simulink model "ctrl_typeA"  (R2016b)
settings: Solver=ode45  StartTime=0.0  StopTime=12.0  RelTol=1e-3  EnableMultiTasking=on
undefined symbols (not defined in the file): cMat_BF, cMat_IM, cMat_MN, cMat_TM, gain_actBFGAS, gain_actBFL, gain_actBFP, gain_actBFR, gain_actBFT, gain_actBFV, gain_actBFY, gain_actF0GAS, gain_actF1GAS, gain_actF2GAS, gain_actF3GAS, gain_actIML, gain_actIMP, gain_actIMR, gain_actIMT, gain_actIMV, gain_actIMY, gain_actIPL, gain_actIPT, gain_actIPY, gain_actMNL, gain_actMNP, gain_actMNR, gain_actMNT, gain_actMNV, gain_actMNY, gain_actTML, gain_actTMP, gain_actTMY, gainBFGAS, gainBFL, gainBFP, gainBFR, gainBFT, gainBFV, gainBFY, gainF0GAS, gainF1GAS, gainF2GAS, gainF3GAS, gainHieBFP, gainHieBFR, gainHieBFY, gainHieIML, gainHieIMP, gainHieIMY, gainHieIPL, gainHieIPY, gainHieMNL, gainHieMNP, gainHieMNY, gainIML, gainIMP, gainIMR, gainIMT, gainIMV ... (+24)
libraries: cstblocks x54
(part 1 of 2)
settings Model: Creator=kokioktm  LastModifiedBy=miyo
settings DataIOCC: LimitDataPoints=on  SaveFormat=Array
settings OptimizationCC: LifeSpan=inf
settings DebuggingCC: SFUnexpectedBacktrackingDiag=warning  SFNoUnconditionalDefaultTransitionDiag=warning  SFExecutionAtInitializationDiag=none
settings HardwareCC: ProdBitPerPointer=32  ProdBitPerSizeT=32  ProdBitPerPtrDiffT=32  ProdLargestAtomicFloat=None  ProdIntDivRoundTo=Undefined  ProdEndianess=Unspecified  ProdWordSize=32  ProdHWDeviceType=32-bit Generic
settings ModelReferenceCC: PropagateSignalLabelsOutOfModel=off
settings GRTTargetCC: TargetLangStandard=C89/C90 (ANSI)  GeneratePreprocessorConditionals=Disable all
settings ConfigComp: CovMetricSettings=dw  CovHtmlReporting=on  CovSaveCumulativeToWorkspaceVar=on  CovSaveSingleToWorkspaceVar=on  CovExternalEMLEnable=off  CovSFcnEnable=off

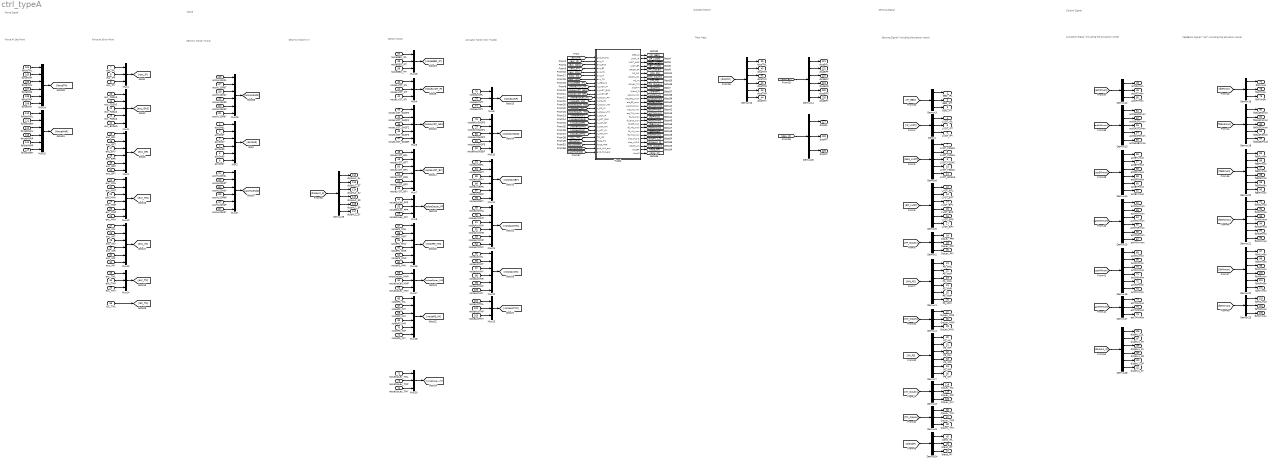
== system ctrl_typeA ==
  note: Actuator Noise
      | (only TypeA)
  note: Force
      | at Error Point
  note: Sensor Noise
  note: Seismic Noise
      | (m/s/s)
  note: Noise
  note: Seismic Noise
      | (m)
  note: Sensing Signal
      | (including the
      | sensor noise)
  note: FeedBack Signal
      | ("not" including the
      | actuation noise)
  note: Actuation Signal
      | (including the
      | actuation noise)
  note: Force
      | At Set Point
  note: Force Signal
  note: Control Signal
  note: Sensing Signal
  note: Test Mass
  note: Isolated Motion
  accGndL : Inport
  accGndT : Inport  Port=2
  accGndV : Inport  Port=3
  accGndR : Inport  Port=4
  accGndP : Inport  Port=5
  accGndY : Inport  Port=6
  exc_IPL : Inport  Port=7
  exc_IPT : Inport  Port=8
  exc_IPY : Inport  Port=9
  exc_F0GAS : Inport  Port=10
  exc_F1GAS : Inport  Port=11
  exc_F2GAS : Inport  Port=12
  exc_F3GAS : Inport  Port=13
  exc_BFGAS : Inport  Port=14
  exc_BFL : Inport  Port=15
  exc_BFT : Inport  Port=16
  exc_BFV : Inport  Port=17
  exc_BFR : Inport  Port=18
  exc_BFP : Inport  Port=19
  exc_BFY : Inport  Port=20
  exc_MNL : Inport  Port=21
  exc_MNT : Inport  Port=22
  exc_MNV : Inport  Port=23
  exc_MNR : Inport  Port=24
  exc_MNP : Inport  Port=25
  exc_MNY : Inport  Port=26
  exc_IML : Inport  Port=27
  exc_IMT : Inport  Port=28
  exc_IMV : Inport  Port=29
  exc_IMR : Inport  Port=30
  exc_IMP : Inport  Port=31
  exc_IMY : Inport  Port=32
  exc_TML : Inport  Port=33
  exc_TMP : Inport  Port=34
  exc_TMY : Inport  Port=35
  ISC_TML : Inport  Port=36
  noiseGEO_IPL : Inport  Port=37
  noiseGEO_IPT : Inport  Port=38
  noiseGEO_IPY : Inport  Port=39
  noiseLVDT_IPL : Inport  Port=40
  noiseLVDT_IPT : Inport  Port=41
  noiseLVDT_IPY : Inport  Port=42
  noiseLVDT_GASF0 : Inport  Port=43
  noiseLVDT_GASF1 : Inport  Port=44
  noiseLVDT_GASF2 : Inport  Port=45
  noiseLVDT_GASF3 : Inport  Port=46
  noiseLVDT_GASBF : Inport  Port=47
  noiseLVDT_BFL : Inport  Port=48
  noiseLVDT_BFT : Inport  Port=49
  noiseLVDT_BFV : Inport  Port=50
  noiseLVDT_BFR : Inport  Port=51
  noiseLVDT_BFP : Inport  Port=52
  noiseLVDT_BFY : Inport  Port=53
  noiseOpLev_PFR : Inport  Port=54
  noiseOpLev_PFP : Inport  Port=55
  noiseOpLev_PFY : Inport  Port=56
  noisePS_MNL : Inport  Port=57
  noisePS_MNT : Inport  Port=58
  noisePS_MNV : Inport  Port=59
  noisePS_MNR : Inport  Port=60
  noisePS_MNP : Inport  Port=61
  noisePS_MNY : Inport  Port=62
  noiseOpLev_MNR : Inport  Port=63
  noiseOpLev_MNP : Inport  Port=64
  noiseOpLev_MNY : Inport  Port=65
  noisePS_IML : Inport  Port=66
  noisePS_IMT : Inport  Port=67
  noisePS_IMV : Inport  Port=68
  noisePS_IMR : Inport  Port=69
  noisePS_IMP : Inport  Port=70
  noisePS_IMY : Inport  Port=71
  noiseOpLev_TML : Inport  Port=72
  noiseOpLev_TMP : Inport  Port=73
  noiseOpLev_TMY : Inport  Port=74
  noiseActIPL : Inport  Port=75
  noiseActIPT : Inport  Port=76
  noiseActIPY : Inport  Port=77
  noiseActGASF0 : Inport  Port=78
  noiseActGASF1 : Inport  Port=79
  noiseActGASF2 : Inport  Port=80
  noiseActGASF3 : Inport  Port=81
  noiseActGASBF : Inport  Port=82
  noiseActBFL : Inport  Port=83
  noiseActBFT : Inport  Port=84
  noiseActBFV : Inport  Port=85
  noiseActBFR : Inport  Port=86
  noiseActBFP : Inport  Port=87
  noiseActBFY : Inport  Port=88
  noiseActMNL : Inport  Port=89
  noiseActMNT : Inport  Port=90
  noiseActMNV : Inport  Port=91
  noiseActMNR : Inport  Port=92
  noiseActMNP : Inport  Port=93
  noiseActMNY : Inport  Port=94
  noiseActIML : Inport  Port=95
  noiseActIMT : Inport  Port=96
  noiseActIMV : Inport  Port=97
  noiseActIMR : Inport  Port=98
  noiseActIMP : Inport  Port=99
  noiseActIMY : Inport  Port=100
  noiseActTML : Inport  Port=101
  noiseActTMP : Inport  Port=102
  noiseActTMY : Inport  Port=103
  forceTML : Inport  Port=104
  forceTMT : Inport  Port=105
  forceTMV : Inport  Port=106
  forceTMR : Inport  Port=107
  forceTMP : Inport  Port=108
  forceTMY : Inport  Port=109
  forceMNRL : Inport  Port=110
  forceMNRT : Inport  Port=111
  forceMNRV : Inport  Port=112
  forceMNRR : Inport  Port=113
  forceMNRP : Inport  Port=114
  forceMNRY : Inport  Port=115
  accHL1GndL : Inport  Port=116
  accHL1GndT : Inport  Port=117
  accHL1GndV : Inport  Port=118
  accHL1GndR : Inport  Port=119
  accHL1GndP : Inport  Port=120
  accHL1GndY : Inport  Port=121
  accHL2GndL : Inport  Port=122
  accHL2GndT : Inport  Port=123
  accHL2GndV : Inport  Port=124
  accHL2GndR : Inport  Port=125
  accHL2GndP : Inport  Port=126
  accHL2GndY : Inport  Port=127
  Demux{,2..4,8..9,12,17..18,23..25} (12 alike) : Demux  Outputs=3
  Demux{1,5,7,10..11,14..16,20..22,28..29} (13 alike) : Demux  Outputs=6
  Demux13 : Demux  Outputs=5
  Demux19 : Demux  Outputs=5
  Demux6 : Demux  Outputs=5
  Mux{1,4,8..9,14..15,17,20,23} (9 alike) : Mux  Inputs=3
  Mux10 : Mux  Inputs=5
  Mux{2..3,7,11..13,16,18,21..22,24..27} (14 alike) : Mux  Inputs=6
  Mux5 : Mux  Inputs=5
  Mux6 : Mux  Inputs=5
  TypeA : Subsystem
  GEO_IPL : Outport
  GEO_IPT : Outport  Port=2
  GEO_IPY : Outport  Port=3
  LVDT_IPL : Outport  Port=4
  LVDT_IPT : Outport  Port=5
  LVDT_IPY : Outport  Port=6
  LVDT_F0GAS : Outport  Port=7
  LVDT_F1GAS : Outport  Port=8
  LVDT_F2GAS : Outport  Port=9
  LVDT_F3GAS : Outport  Port=10
  LVDT_BFGAS : Outport  Port=11
  LVDT_BFL : Outport  Port=12
  LVDT_BFT : Outport  Port=13
  LVDT_BFV : Outport  Port=14
  LVDT_BFR : Outport  Port=15
  LVDT_BFP : Outport  Port=16
  LVDT_BFY : Outport  Port=17
  OpLev_PFR : Outport  Port=18
  OpLev_PFP : Outport  Port=19
  OpLev_PFY : Outport  Port=20
  PS_MNL : Outport  Port=21
  PS_MNT : Outport  Port=22
  PS_MNV : Outport  Port=23
  PS_MNR : Outport  Port=24
  PS_MNP : Outport  Port=25
  PS_MNY : Outport  Port=26
  OpLev_MNR : Outport  Port=27
  OpLev_MNP : Outport  Port=28
  OpLev_MNY : Outport  Port=29
  PS_IML : Outport  Port=30
  PS_IMT : Outport  Port=31
  PS_IMV : Outport  Port=32
  PS_IMR : Outport  Port=33
  PS_IMP : Outport  Port=34
  PS_IMY : Outport  Port=35
  OpLev_TML : Outport  Port=36
  OpLev_TMP : Outport  Port=37
  OpLev_TMY : Outport  Port=38
  dispTML : Outport  Port=39
  dispTMT : Outport  Port=40
  dispTMV : Outport  Port=41
  dispTMR : Outport  Port=42
  dispTMP : Outport  Port=43
  dispTMY : Outport  Port=44
  blend_IPL : Outport  Port=45
  blend_IPT : Outport  Port=46
  blend_IPY : Outport  Port=47
  actIPLmon : Outport  Port=48
  actIPTmon : Outport  Port=49
  actIPYmon : Outport  Port=50
  actGASF0mon : Outport  Port=51
  actGASF1mon : Outport  Port=52
  actGASF2mon : Outport  Port=53
  actGASF3mon : Outport  Port=54
  actGASBFmon : Outport  Port=55
  actBFLmon : Outport  Port=56
  actBFTmon : Outport  Port=57
  actBFVmon : Outport  Port=58
  actBFRmon : Outport  Port=59
  actBFPmon : Outport  Port=60
  actBFYmon : Outport  Port=61
  actMNLmon : Outport  Port=62
  actMNTmon : Outport  Port=63
  actMNVmon : Outport  Port=64
  actMNRmon : Outport  Port=65
  actMNPmon : Outport  Port=66
  actMNYmon : Outport  Port=67
  actIMLmon : Outport  Port=68
  actIMTmon : Outport  Port=69
  actIMVmon : Outport  Port=70
  actIMRmon : Outport  Port=71
  actIMPmon : Outport  Port=72
  actIMYmon : Outport  Port=73
  actTMLmon : Outport  Port=74
  actTMPmon : Outport  Port=75
  actTMYmon : Outport  Port=76
  fbIPLmon : Outport  Port=77
  fbIPTmon : Outport  Port=78
  fbIPYmon : Outport  Port=79
  fbGASF0mon : Outport  Port=80
  fbGASF1mon : Outport  Port=81
  fbGASF2mon : Outport  Port=82
  fbGASF3mon : Outport  Port=83
  fbGASBFmon : Outport  Port=84
  fbBFLmon : Outport  Port=85
  fbBFTmon : Outport  Port=86
  fbBFVmon : Outport  Port=87
  fbBFRmon : Outport  Port=88
  fbBFPmon : Outport  Port=89
  fbBFYmon : Outport  Port=90
  fbMNLmon : Outport  Port=91
  fbMNTmon : Outport  Port=92
  fbMNVmon : Outport  Port=93
  fbMNRmon : Outport  Port=94
  fbMNPmon : Outport  Port=95
  fbMNYmon : Outport  Port=96
  fbIMLmon : Outport  Port=97
  fbIMTmon : Outport  Port=98
  fbIMVmon : Outport  Port=99
  fbIMRmon : Outport  Port=100
  fbIMPmon : Outport  Port=101
  fbIMYmon : Outport  Port=102
  fbTMLmon : Outport  Port=103
  fbTMPmon : Outport  Port=104
  fbTMYmon : Outport  Port=105
  dispHL1_3L : Outport  Port=106
  dispHL1_3T : Outport  Port=107
  dispHL1_3V : Outport  Port=108
  dispHL1_3R : Outport  Port=109
  dispHL1_3P : Outport  Port=110
  dispHL1_3Y : Outport  Port=111
  dispHL2_3L : Outport  Port=112
  dispHL2_3T : Outport  Port=113
  dispHL2_3V : Outport  Port=114
  dispHL2_3R : Outport  Port=115
  dispHL2_3P : Outport  Port=116
  dispHL2_3Y : Outport  Port=117
  OpLev_IML : Outport  Port=118
  OpLev_IMP : Outport  Port=119
  OpLev_IMY : Outport  Port=120
  dispBFL : Outport  Port=121
  dispBFT : Outport  Port=122
  dispBFV : Outport  Port=123
  dispBFR : Outport  Port=124
  dispBFP : Outport  Port=125
  dispBFY : Outport  Port=126
  dispIPL : Outport  Port=127
  dispIPT : Outport  Port=128
  dispIPY : Outport  Port=129
  wires:
  [accGnd] -> TypeA/1(gnd_2F_acc)
  accGndT/1 -> Mux2/2
  accGndL/1 -> Mux2/1
  accGndV/1 -> Mux2/3
  accGndR/1 -> Mux2/4
  accGndP/1 -> Mux2/5
  accGndY/1 -> Mux2/6
  Mux2/1 -> [accGnd]
  exc_IPL/1 -> Mux1/1
  exc_IPT/1 -> Mux1/2
  exc_IPY/1 -> Mux1/3
  Mux1/1 -> [exc_IP]
  [exc_IP] -> TypeA/2(exc_IP)
  exc_F0GAS/1 -> Mux5/1
  exc_F1GAS/1 -> Mux5/2
  exc_F2GAS/1 -> Mux5/3
  exc_F3GAS/1 -> Mux5/4
  exc_BFGAS/1 -> Mux5/5
  Mux5/1 -> [exc_GAS]
  [exc_GAS] -> TypeA/3(exc_GAS)
  exc_BFT/1 -> Mux3/2
  exc_BFL/1 -> Mux3/1
  exc_BFV/1 -> Mux3/3
  exc_BFR/1 -> Mux3/4
  exc_BFP/1 -> Mux3/5
  exc_BFY/1 -> Mux3/6
  Mux3/1 -> [exc_BF]
  [exc_BF] -> TypeA/4(exc_BF)
  TypeA/2(LVDT_IP) -> [IP_LVDT]
  TypeA/3(LVDT_GAS) -> [GAS_LVDT]
  TypeA/4(LVDT_BF) -> [BF_LVDT]
  TypeA/10(dispTM) -> [dispTM]
  TypeA/5(OPLEV_PF) -> [PF_OpLev]
  [IP_LVDT] -> Demux/1
  Demux/1 -> LVDT_IPL/1
  Demux/2 -> LVDT_IPT/1
  Demux/3 -> LVDT_IPY/1
  [GAS_LVDT] -> Demux6/1
  Demux6/1 -> LVDT_F0GAS/1
  Demux6/2 -> LVDT_F1GAS/1
  Demux6/3 -> LVDT_F2GAS/1
  Demux6/4 -> LVDT_F3GAS/1
  Demux6/5 -> LVDT_BFGAS/1
  [BF_LVDT] -> Demux5/1
  Demux5/1 -> LVDT_BFL/1
  Demux5/2 -> LVDT_BFT/1
  Demux5/3 -> LVDT_BFV/1
  Demux5/4 -> LVDT_BFR/1
  Demux5/5 -> LVDT_BFP/1
  Demux5/6 -> LVDT_BFY/1
  Demux1/1 -> PS_MNL/1
  Demux1/2 -> PS_MNT/1
  Demux1/3 -> PS_MNV/1
  Demux1/4 -> PS_MNR/1
  Demux1/5 -> PS_MNP/1
  Demux1/6 -> PS_MNY/1
  [MN_PS] -> Demux1/1
  [PF_OpLev] -> Demux2/1
  Demux2/2 -> OpLev_PFP/1
  Demux2/3 -> OpLev_PFY/1
  noiseLVDT_IPL/1 -> Mux4/1
  noiseLVDT_IPT/1 -> Mux4/2
  noiseLVDT_IPY/1 -> Mux4/3
  Mux4/1 -> [noiseLVDT_IP]
  noiseLVDT_GASF0/1 -> Mux6/1
  noiseLVDT_GASF1/1 -> Mux6/2
  noiseLVDT_GASF2/1 -> Mux6/3
  noiseLVDT_GASF3/1 -> Mux6/4
  noiseLVDT_GASBF/1 -> Mux6/5
  Mux6/1 -> [noiseLVDT_GAS]
  noiseLVDT_BFT/1 -> Mux7/2
  noiseLVDT_BFL/1 -> Mux7/1
  noiseLVDT_BFV/1 -> Mux7/3
  noiseLVDT_BFR/1 -> Mux7/4
  noiseLVDT_BFP/1 -> Mux7/5
  noiseLVDT_BFY/1 -> Mux7/6
  Mux7/1 -> [noiseLVDT_BF]
  noiseOpLev_PFR/1 -> Mux8/1
  noiseOpLev_PFP/1 -> Mux8/2
  Mux8/1 -> [noiseOpLev_PF]
  [noiseLVDT_IP] -> TypeA/9(n_LVDT_IP)
  [noiseLVDT_GAS] -> TypeA/10(n_LVDT_GAS)
  [noiseOpLev_PF] -> TypeA/12(n_OpLev_PF)
  [noiseLVDT_BF] -> TypeA/11(n_LVDT_BF)
  noiseActIPL/1 -> Mux9/1
  noiseActIPT/1 -> Mux9/2
  noiseActIPY/1 -> Mux9/3
  Mux9/1 -> [noiseActIP]
  noiseActGASF0/1 -> Mux10/1
  noiseActGASF1/1 -> Mux10/2
  noiseActGASF2/1 -> Mux10/3
  noiseActGASF3/1 -> Mux10/4
  noiseActGASBF/1 -> Mux10/5
  Mux10/1 -> [noiseActGAS]
  noiseActBFT/1 -> Mux11/2
  noiseActBFL/1 -> Mux11/1
  noiseActBFV/1 -> Mux11/3
  noiseActBFR/1 -> Mux11/4
  noiseActBFP/1 -> Mux11/5
  noiseActBFY/1 -> Mux11/6
  Mux11/1 -> [noiseActBF]
  [noiseActGAS] -> TypeA/18(n_ACT_GAS)
  [noiseActBF] -> TypeA/19(n_ACT_BF)
  [noiseActIP] -> TypeA/17(n_ACT_IP)
  [exc_MN] -> TypeA/5(exc_MN)
  [exc_TM] -> TypeA/7(exc_TM)
  [exc_IM] -> TypeA/6(exc_IM)
  exc_MNT/1 -> Mux12/2
  exc_MNL/1 -> Mux12/1
  exc_MNV/1 -> Mux12/3
  exc_MNR/1 -> Mux12/4
  exc_MNP/1 -> Mux12/5
  exc_MNY/1 -> Mux12/6
  Mux12/1 -> [exc_MN]
  exc_IMT/1 -> Mux13/2
  exc_IML/1 -> Mux13/1
  exc_IMV/1 -> Mux13/3
  exc_IMR/1 -> Mux13/4
  exc_IMP/1 -> Mux13/5
  exc_IMY/1 -> Mux13/6
  Mux13/1 -> [exc_IM]
  exc_TML/1 -> Mux14/1
  exc_TMP/1 -> Mux14/2
  exc_TMY/1 -> Mux14/3
  Mux14/1 -> [exc_TM]
  noiseGEO_IPL/1 -> Mux15/1
  noiseGEO_IPT/1 -> Mux15/2
  noiseGEO_IPY/1 -> Mux15/3
  Mux15/1 -> [noiseGEO_IP]
  [noiseGEO_IP] -> TypeA/8(n_GEO_IP)
  noiseOpLev_PFY/1 -> Mux8/3
  noisePS_MNT/1 -> Mux16/2
  noisePS_MNL/1 -> Mux16/1
  noisePS_MNV/1 -> Mux16/3
  noisePS_MNR/1 -> Mux16/4
  noisePS_MNP/1 -> Mux16/5
  noisePS_MNY/1 -> Mux16/6
  Mux16/1 -> [noisePS_MN]
  noiseOpLev_MNR/1 -> Mux17/1
  noiseOpLev_MNP/1 -> Mux17/2
  Mux17/1 -> [noiseOpLev_MN]
  noiseOpLev_MNY/1 -> Mux17/3
  noisePS_IMT/1 -> Mux18/2
  noisePS_IML/1 -> Mux18/1
  noisePS_IMV/1 -> Mux18/3
  noisePS_IMR/1 -> Mux18/4
  noisePS_IMP/1 -> Mux18/5
  noisePS_IMY/1 -> Mux18/6
  Mux18/1 -> [noisePS_IM]
  noiseOpLev_TMP/1 -> Mux20/2
  noiseOpLev_TMY/1 -> Mux20/3
  Mux20/1 -> [noiseOpLev_TM]
  [noisePS_MN] -> TypeA/13(n_PS_MN)
  [noisePS_IM] -> TypeA/15(n_PS_IM)
  [noiseOpLev_MN] -> TypeA/14(n_OpLev_MN)
  [noiseOpLev_TM] -> TypeA/16(n_OpLev_TM)
  noiseActMNT/1 -> Mux21/2
  noiseActMNL/1 -> Mux21/1
  noiseActMNV/1 -> Mux21/3
  noiseActMNR/1 -> Mux21/4
  noiseActMNP/1 -> Mux21/5
  noiseActMNY/1 -> Mux21/6
  Mux21/1 -> [noiseActMN]
  noiseActIMT/1 -> Mux22/2
  noiseActIML/1 -> Mux22/1
  noiseActIMV/1 -> Mux22/3
  noiseActIMR/1 -> Mux22/4
  noiseActIMP/1 -> Mux22/5
  noiseActIMY/1 -> Mux22/6
  Mux22/1 -> [noiseActIM]
  noiseActTML/1 -> Mux23/1
  noiseActTMP/1 -> Mux23/2
  noiseActTMY/1 -> Mux23/3
  Mux23/1 -> [noiseActTM]
  forceTMT/1 -> Mux24/2
  forceTML/1 -> Mux24/1
  forceTMV/1 -> Mux24/3
  forceTMR/1 -> Mux24/4
  forceTMP/1 -> Mux24/5
  forceTMY/1 -> Mux24/6
  Mux24/1 -> [forceTM]
  ISC_TML/1 -> [ISC_TM]
  [noiseActMN] -> TypeA/20(n_ACT_MN)
  [noiseActTM] -> TypeA/22(n_ACT_TM)
  [noiseActIM] -> TypeA/21(n_ACT_IM)
  [forceTM] -> TypeA/24(force_TM)
  [ISC_TM] -> TypeA/23(TM_ISC)
  [IP_GEO] -> Demux3/1
  Demux3/1 -> GEO_IPL/1
  Demux3/2 -> GEO_IPT/1
  Demux3/3 -> GEO_IPY/1
  TypeA/1(GEO_IP) -> [IP_GEO]
  Demux2/1 -> OpLev_PFR/1
  TypeA/8(PS_IM) -> [IM_PS]
  TypeA/7(OPLEV_MN) -> [MN_OpLev]
  TypeA/6(PS_MN) -> [MN_PS]
  TypeA/9(OPLEV_TM) -> [TM_OpLev]
  TypeA/19(fb_GAS_mon) -> [fbGASmon]
  TypeA/13(act_GAS_mon) -> [actGASmon]
  TypeA/18(fb_IP_mon) -> [fbIPmon]
  TypeA/23(fb_TM_mon) -> [fbTMmon]
  TypeA/21(fb_MN_mon) -> [fbMNmon]
  TypeA/12(act_IP_mon) -> [actIPmon]
  TypeA/16(act_IM_mon) -> [actIMmon]
  TypeA/11(blend_IP) -> [blendIP]
  TypeA/22(fb_IM_mon) -> [fbIMmon]
  TypeA/15(act_MN_mon) -> [actMNmon]
  TypeA/17(act_TM_mon) -> [actTMmon]
  TypeA/14(act_BF_mon) -> [actBFmon]
  TypeA/20(fb_BF_mon) -> [fbBFmon]
  [MN_OpLev] -> Demux4/1
  Demux4/2 -> OpLev_MNP/1
  Demux4/3 -> OpLev_MNY/1
  Demux4/1 -> OpLev_MNR/1
  Demux7/1 -> PS_IML/1
  Demux7/2 -> PS_IMT/1
  Demux7/3 -> PS_IMV/1
  Demux7/4 -> PS_IMR/1
  Demux7/5 -> PS_IMP/1
  Demux7/6 -> PS_IMY/1
  [IM_PS] -> Demux7/1
  [TM_OpLev] -> Demux9/1
  Demux10/1 -> dispTML/1
  Demux10/2 -> dispTMT/1
  Demux10/3 -> dispTMV/1
  Demux10/4 -> dispTMR/1
  Demux10/5 -> dispTMP/1
  Demux10/6 -> dispTMY/1
  [dispTM] -> Demux10/1
  [actIPmon] -> Demux12/1
  Demux12/1 -> actIPLmon/1
  Demux12/2 -> actIPTmon/1
  Demux12/3 -> actIPYmon/1
  [actGASmon] -> Demux13/1
  Demux13/1 -> actGASF0mon/1
  Demux13/2 -> actGASF1mon/1
  Demux13/3 -> actGASF2mon/1
  Demux13/4 -> actGASF3mon/1
  Demux13/5 -> actGASBFmon/1
  [actBFmon] -> Demux14/1
  Demux14/1 -> actBFLmon/1
  Demux14/2 -> actBFTmon/1
  Demux14/3 -> actBFVmon/1
  Demux14/4 -> actBFRmon/1
  Demux14/5 -> actBFPmon/1
  Demux14/6 -> actBFYmon/1
  [actMNmon] -> Demux15/1
  Demux15/1 -> actMNLmon/1
  Demux15/2 -> actMNTmon/1
  Demux15/3 -> actMNVmon/1
  Demux15/4 -> actMNRmon/1
  Demux15/5 -> actMNPmon/1
  Demux15/6 -> actMNYmon/1
  [actIMmon] -> Demux16/1
  Demux16/1 -> actIMLmon/1
  Demux16/2 -> actIMTmon/1
  Demux16/3 -> actIMVmon/1
  Demux16/4 -> actIMRmon/1
  Demux16/5 -> actIMPmon/1
  Demux16/6 -> actIMYmon/1
  [actTMmon] -> Demux17/1
  Demux17/2 -> actTMPmon/1
  Demux17/3 -> actTMYmon/1
  Demux17/1 -> actTMLmon/1
  [fbIPmon] -> Demux18/1
  Demux18/1 -> fbIPLmon/1
  Demux18/2 -> fbIPTmon/1
  Demux18/3 -> fbIPYmon/1
  [fbGASmon] -> Demux19/1
  Demux19/1 -> fbGASF0mon/1
  Demux19/2 -> fbGASF1mon/1
  Demux19/3 -> fbGASF2mon/1
  Demux19/4 -> fbGASF3mon/1
  Demux19/5 -> fbGASBFmon/1
  [fbBFmon] -> Demux20/1
  Demux20/1 -> fbBFLmon/1
  Demux20/2 -> fbBFTmon/1
  Demux20/3 -> fbBFVmon/1
  Demux20/4 -> fbBFRmon/1
  Demux20/5 -> fbBFPmon/1
  Demux20/6 -> fbBFYmon/1
  [fbMNmon] -> Demux21/1
  Demux21/1 -> fbMNLmon/1
  Demux21/2 -> fbMNTmon/1
  Demux21/3 -> fbMNVmon/1
  Demux21/4 -> fbMNRmon/1
  Demux21/5 -> fbMNPmon/1
  Demux21/6 -> fbMNYmon/1
  [fbIMmon] -> Demux22/1
  Demux22/1 -> fbIMLmon/1
  Demux22/2 -> fbIMTmon/1
  Demux22/3 -> fbIMVmon/1
  Demux22/4 -> fbIMRmon/1
  Demux22/5 -> fbIMPmon/1
  Demux22/6 -> fbIMYmon/1
  [fbTMmon] -> Demux23/1
  Demux23/2 -> fbTMPmon/1
  Demux23/3 -> fbTMYmon/1
  Demux23/1 -> fbTMLmon/1
  Demux24/1 -> blend_IPL/1
  [blendIP] -> Demux24/1
  Demux24/2 -> blend_IPT/1
  Demux24/3 -> blend_IPY/1
  forceMNRR/1 -> Mux25/4
  forceMNRP/1 -> Mux25/5
  forceMNRL/1 -> Mux25/1
  forceMNRT/1 -> Mux25/2
  Mux25/1 -> [forceMNR]
  forceMNRV/1 -> Mux25/3
  forceMNRY/1 -> Mux25/6
  [forceMNR] -> TypeA/25(force_MNR)
  noiseOpLev_TML/1 -> Mux20/1
  Demux9/1 -> OpLev_TML/1
  Demux9/2 -> OpLev_TMP/1
  Demux9/3 -> OpLev_TMY/1
  TypeA/24(disp_HL1-3) -> [dispHL1_3]
  TypeA/25(disp_HL2-3) -> [dispHL2_3]
  Demux28/3 -> dispHL1_3V/1
  Demux28/1 -> dispHL1_3L/1
  Demux28/4 -> dispHL1_3R/1
  Demux28/2 -> dispHL1_3T/1
  Demux28/5 -> dispHL1_3P/1
  [dispHL1_3] -> Demux28/1
  Demux28/6 -> dispHL1_3Y/1
  Demux29/6 -> dispHL2_3Y/1
  [dispHL2_3] -> Demux29/1
  Demux29/1 -> dispHL2_3L/1
  Demux29/2 -> dispHL2_3T/1
  Demux29/5 -> dispHL2_3P/1
  Demux29/3 -> dispHL2_3V/1
  Demux29/4 -> dispHL2_3R/1
  accHL1GndP/1 -> Mux26/5
  accHL1GndL/1 -> Mux26/1
  accHL1GndR/1 -> Mux26/4
  accHL1GndY/1 -> Mux26/6
  Mux26/1 -> [accHLGnd1]
  accHL1GndV/1 -> Mux26/3
  accHL1GndT/1 -> Mux26/2
  [accHLGnd1] -> TypeA/26(gnd_HL1_acc)
  accHL2GndV/1 -> Mux27/3
  accHL2GndT/1 -> Mux27/2
  accHL2GndY/1 -> Mux27/6
  Mux27/1 -> [accHLGnd2]
  accHL2GndR/1 -> Mux27/4
  accHL2GndL/1 -> Mux27/1
  accHL2GndP/1 -> Mux27/5
  [accHLGnd2] -> TypeA/27(gnd_HL2_acc)
  TypeA/26(OPLEV_IM) -> [IM_OpLev]
  [IM_OpLev] -> Demux8/1
  Demux8/1 -> OpLev_IML/1
  Demux8/2 -> OpLev_IMP/1
  Demux8/3 -> OpLev_IMY/1
  TypeA/27(dispBF) -> [disp_BF]
  Demux11/1 -> dispBFL/1
  Demux11/2 -> dispBFT/1
  Demux11/3 -> dispBFV/1
  Demux11/4 -> dispBFR/1
  Demux11/5 -> dispBFP/1
  Demux11/6 -> dispBFY/1
  [disp_BF] -> Demux11/1
  TypeA/28(dispIP) -> [disp_IP]
  Demux25/1 -> dispIPL/1
  Demux25/2 -> dispIPT/1
  [disp_IP] -> Demux25/1
  Demux25/3 -> dispIPY/1

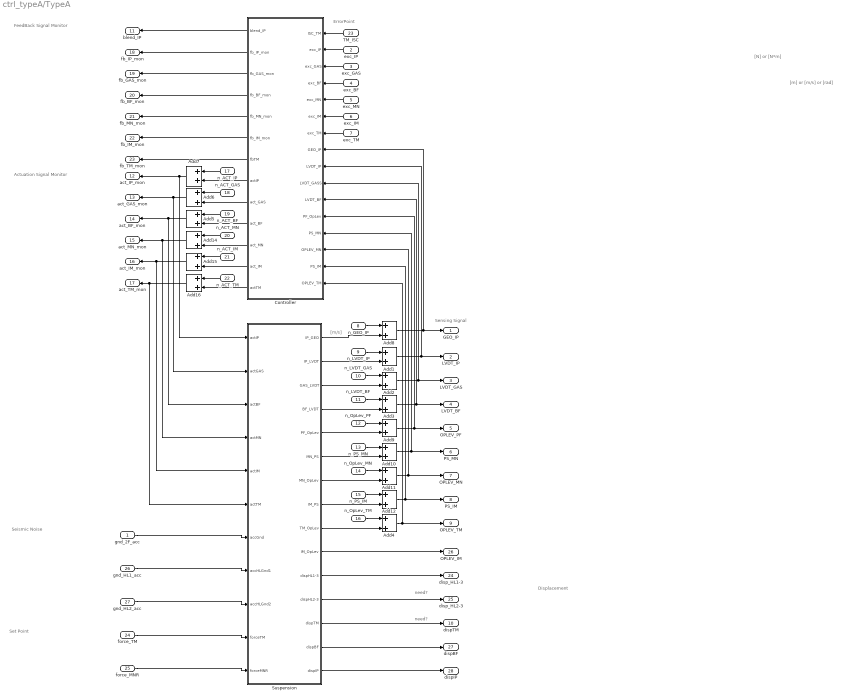
== system ctrl_typeA/TypeA ==
  note: [m] or [m/s] or [rad]
  note: [N] or [N*m]
  note: Sensing Signal
  note: Displacement
  note: Seismic
      | Noise
  note: Set Point
  note: Actuation Signal
      | Monitor
  note: FeedBack Signal
      | Monitor
  note: ErrorPoint
  note: [m/s]
  note: need?
  note: need?
  gnd_2F_acc : Inport
  exc_IP : Inport  Port=2
  exc_GAS : Inport  Port=3
  exc_BF : Inport  Port=4
  exc_MN : Inport  Port=5
  exc_IM : Inport  Port=6
  exc_TM : Inport  Port=7
  n_GEO_IP : Inport  Port=8
  n_LVDT_IP : Inport  Port=9
  n_LVDT_GAS : Inport  Port=10
  n_LVDT_BF : Inport  Port=11
  n_OpLev_PF : Inport  Port=12
  n_PS_MN : Inport  Port=13
  n_OpLev_MN : Inport  Port=14
  n_PS_IM : Inport  Port=15
  n_OpLev_TM : Inport  Port=16
  n_ACT_IP : Inport  Port=17
  n_ACT_GAS : Inport  Port=18
  n_ACT_BF : Inport  Port=19
  n_ACT_MN : Inport  Port=20
  n_ACT_IM : Inport  Port=21
  n_ACT_TM : Inport  Port=22
  TM_ISC : Inport  Port=23
  force_TM : Inport  Port=24
  force_MNR : Inport  Port=25
  gnd_HL1_acc : Inport  Port=26
  gnd_HL2_acc : Inport  Port=27
  Add{1..12,14..16} (15 alike) : Sum
  Controller : Subsystem
  Suspension : Subsystem
  GEO_IP : Outport
  LVDT_IP : Outport  Port=2
  LVDT_GAS : Outport  Port=3
  LVDT_BF : Outport  Port=4
  OPLEV_PF : Outport  Port=5
  PS_MN : Outport  Port=6
  OPLEV_MN : Outport  Port=7
  PS_IM : Outport  Port=8
  OPLEV_TM : Outport  Port=9
  dispTM : Outport  Port=10
  blend_IP : Outport  Port=11
  act_IP_mon : Outport  Port=12
  act_GAS_mon : Outport  Port=13
  act_BF_mon : Outport  Port=14
  act_MN_mon : Outport  Port=15
  act_IM_mon : Outport  Port=16
  act_TM_mon : Outport  Port=17
  fb_IP_mon : Outport  Port=18
  fb_GAS_mon : Outport  Port=19
  fb_BF_mon : Outport  Port=20
  fb_MN_mon : Outport  Port=21
  fb_IM_mon : Outport  Port=22
  fb_TM_mon : Outport  Port=23
  disp_HL1-3 : Outport  Port=24
  disp_HL2-3 : Outport  Port=25
  OPLEV_IM : Outport  Port=26
  dispBF : Outport  Port=27
  dispIP : Outport  Port=28
  wires:
  Add1/1 -> LVDT_IP/1, Controller/9(LVDT_IP)
  Add3/1 -> LVDT_BF/1, Controller/11(LVDT_BF)
  Add2/1 -> LVDT_GAS/1, Controller/10(LVDT_GASS)
  Suspension/13(dispTM) -> dispTM/1
  Add7/1 -> act_IP_mon/1, Suspension/1(actIP)
  Add5/1 -> act_BF_mon/1, Suspension/3(actBF)
  Add4/1 -> OPLEV_TM/1, Controller/16(OPLEV_TM)
  gnd_2F_acc/1 -> Suspension/7(accGnd)
  Add6/1 -> act_GAS_mon/1, Suspension/2(actGAS)
  exc_GAS/1 -> Controller/3(exc_GAS)
  exc_IP/1 -> Controller/2(exc_IP)
  exc_BF/1 -> Controller/4(exc_BF)
  Controller/4(fb_BF_mon) -> fb_BF_mon/1
  Controller/2(fb_IP_mon) -> fb_IP_mon/1
  Controller/3(fb_GAS_mon) -> fb_GAS_mon/1
  Suspension/2(IP_LVDT) -> Add1/2
  Suspension/3(GAS_LVDT) -> Add2/2
  Suspension/4(BF_LVDT) -> Add3/2
  Suspension/9(TM_OpLev) -> Add4/2
  n_LVDT_IP/1 -> Add1/1
  n_LVDT_GAS/1 -> Add2/1
  n_LVDT_BF/1 -> Add3/1
  n_OpLev_TM/1 -> Add4/1
  Controller/10(act_BF) -> Add5/2
  Controller/8(actIP) -> Add7/2
  Controller/9(act_GAS) -> Add6/2
  n_ACT_IP/1 -> Add7/1
  n_ACT_GAS/1 -> Add6/1
  n_ACT_BF/1 -> Add5/1
  Add8/1 -> GEO_IP/1, Controller/8(GEO_IP)
  n_GEO_IP/1 -> Add8/1
  Suspension/1(IP_GEO) -> Add8/2
  n_OpLev_PF/1 -> Add9/1
  Suspension/5(PF_OpLev) -> Add9/2
  Add9/1 -> OPLEV_PF/1, Controller/12(PF_OpLev)
  n_PS_MN/1 -> Add10/1
  Add10/1 -> PS_MN/1, Controller/13(PS_MN)
  n_OpLev_MN/1 -> Add11/1
  Add11/1 -> OPLEV_MN/1, Controller/14(OPLEV_MN)
  n_PS_IM/1 -> Add12/1
  Add12/1 -> PS_IM/1, Controller/15(PS_IM)
  Suspension/7(MN_OpLev) -> Add11/2
  Suspension/6(MN_PS) -> Add10/2
  Suspension/8(IM_PS) -> Add12/2
  exc_MN/1 -> Controller/5(exc_MN)
  exc_TM/1 -> Controller/7(exc_TM)
  exc_IM/1 -> Controller/6(exc_IM)
  TM_ISC/1 -> Controller/1(ISC_TM)
  n_ACT_MN/1 -> Add14/1
  Add14/1 -> act_MN_mon/1, Suspension/4(actMN)
  Controller/11(act_MN) -> Add14/2
  n_ACT_IM/1 -> Add15/1
  Add15/1 -> act_IM_mon/1, Suspension/5(actIM)
  Controller/12(act_IM) -> Add15/2
  n_ACT_TM/1 -> Add16/1
  Add16/1 -> act_TM_mon/1, Suspension/6(actTM)
  Controller/13(actTM) -> Add16/2
  Controller/1(blend_IP) -> blend_IP/1
  Controller/7(fbTM) -> fb_TM_mon/1
  Controller/5(fb_MN_mon) -> fb_MN_mon/1
  Controller/6(fb_IM_mon) -> fb_IM_mon/1
  force_TM/1 -> Suspension/10(forceTM)
  force_MNR/1 -> Suspension/11(forceMNR)
  Suspension/11(dispHL1-3) -> disp_HL1-3/1
  Suspension/12(dispHL2-3) -> disp_HL2-3/1
  gnd_HL1_acc/1 -> Suspension/8(accHLGnd1)
  gnd_HL2_acc/1 -> Suspension/9(accHLGnd2)
  Suspension/10(IM_OpLev) -> OPLEV_IM/1
  Suspension/14(dispBF) -> dispBF/1
  Suspension/15(dispIP) -> dispIP/1

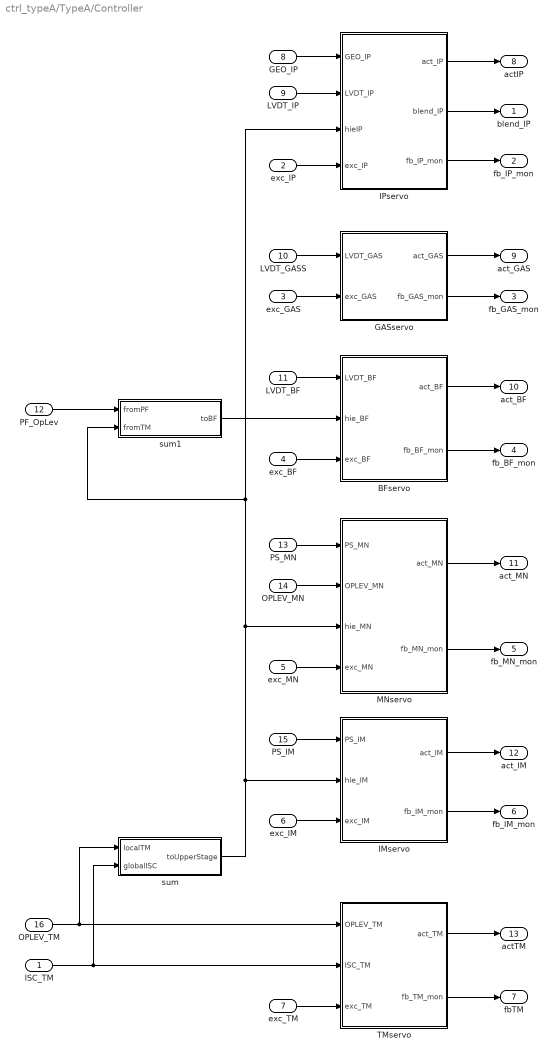
== system ctrl_typeA/TypeA/Controller ==
  ISC_TM : Inport
  exc_IP : Inport  Port=2
  exc_GAS : Inport  Port=3
  exc_BF : Inport  Port=4
  exc_MN : Inport  Port=5
  exc_IM : Inport  Port=6
  exc_TM : Inport  Port=7
  GEO_IP : Inport  Port=8
  LVDT_IP : Inport  Port=9
  LVDT_GASS : Inport  Port=10
  LVDT_BF : Inport  Port=11
  PF_OpLev : Inport  Port=12
  PS_MN : Inport  Port=13
  OPLEV_MN : Inport  Port=14
  PS_IM : Inport  Port=15
  OPLEV_TM : Inport  Port=16
  BFservo : Subsystem
  GASservo : Subsystem
  IMservo : Subsystem
  IPservo : Subsystem
  MNservo : Subsystem
  TMservo : Subsystem
  sum : Subsystem
  sum1 : Subsystem
  blend_IP : Outport
  fb_IP_mon : Outport  Port=2
  fb_GAS_mon : Outport  Port=3
  fb_BF_mon : Outport  Port=4
  fb_MN_mon : Outport  Port=5
  fb_IM_mon : Outport  Port=6
  fbTM : Outport  Port=7
  actIP : Outport  Port=8
  act_GAS : Outport  Port=9
  act_BF : Outport  Port=10
  act_MN : Outport  Port=11
  act_IM : Outport  Port=12
  actTM : Outport  Port=13
  wires:
  LVDT_IP/1 -> IPservo/2(LVDT_IP)
  exc_IP/1 -> IPservo/4(exc_IP)
  IPservo/3(fb_IP_mon) -> fb_IP_mon/1
  IPservo/1(act_IP) -> actIP/1
  GASservo/1(act_GAS) -> act_GAS/1
  GASservo/2(fb_GAS_mon) -> fb_GAS_mon/1
  LVDT_GASS/1 -> GASservo/1(LVDT_GAS)
  exc_GAS/1 -> GASservo/2(exc_GAS)
  LVDT_BF/1 -> BFservo/1(LVDT_BF)
  exc_BF/1 -> BFservo/3(exc_BF)
  BFservo/1(act_BF) -> act_BF/1
  BFservo/2(fb_BF_mon) -> fb_BF_mon/1
  GEO_IP/1 -> IPservo/1(GEO_IP)
  IPservo/2(blend_IP) -> blend_IP/1
  ISC_TM/1 -> sum/2(globalISC), TMservo/2(ISC_TM)
  OPLEV_TM/1 -> sum/1(localTM), TMservo/1(OPLEV_TM)
  exc_TM/1 -> TMservo/3(exc_TM)
  PS_MN/1 -> MNservo/1(PS_MN)
  OPLEV_MN/1 -> MNservo/2(OPLEV_MN)
  exc_MN/1 -> MNservo/4(exc_MN)
  PS_IM/1 -> IMservo/1(PS_IM)
  exc_IM/1 -> IMservo/3(exc_IM)
  TMservo/1(act_TM) -> actTM/1
  TMservo/2(fb_TM_mon) -> fbTM/1
  IMservo/2(fb_IM_mon) -> fb_IM_mon/1
  IMservo/1(act_IM) -> act_IM/1
  MNservo/2(fb_MN_mon) -> fb_MN_mon/1
  MNservo/1(act_MN) -> act_MN/1
  sum/1(toUpperStage) -> sum1/2(fromTM), IPservo/3(hieIP), MNservo/3(hie_MN), IMservo/2(hie_IM)
  sum1/1(toBF) -> BFservo/2(hie_BF)
  PF_OpLev/1 -> sum1/1(fromPF)

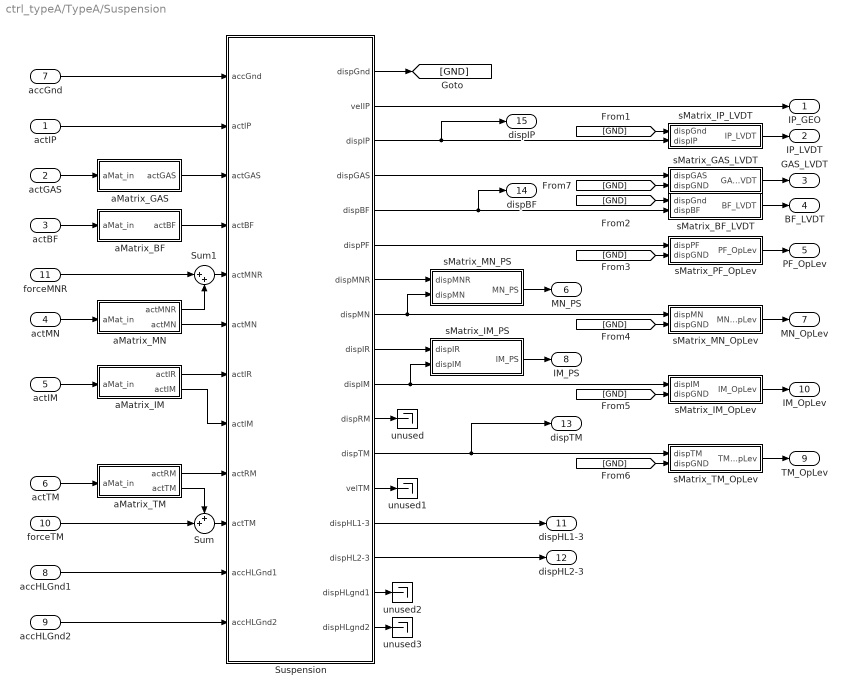
== system ctrl_typeA/TypeA/Suspension ==
  actIP : Inport
  actGAS : Inport  Port=2
  actBF : Inport  Port=3
  actMN : Inport  Port=4
  actIM : Inport  Port=5
  actTM : Inport  Port=6
  accGnd : Inport  Port=7
  accHLGnd1 : Inport  Port=8
  accHLGnd2 : Inport  Port=9
  forceTM : Inport  Port=10
  forceMNR : Inport  Port=11
  Sum : Sum  Inputs=++|
  Sum1 : Sum  Inputs=|++
  Suspension : Subsystem
  aMatrix_BF : Subsystem
  aMatrix_GAS : Subsystem
  aMatrix_IM : Subsystem
  aMatrix_MN : Subsystem
  aMatrix_TM : Subsystem
  sMatrix_BF_LVDT : Subsystem
  sMatrix_GAS_LVDT : Subsystem
  sMatrix_IM_OpLev : Subsystem
  sMatrix_IM_PS : Subsystem
  sMatrix_IP_LVDT : Subsystem
  sMatrix_MN_OpLev : Subsystem
  sMatrix_MN_PS : Subsystem
  sMatrix_PF_OpLev : Subsystem
  sMatrix_TM_OpLev : Subsystem
  unused{,1..3} (4 alike) : Terminator
  IP_GEO : Outport
  IP_LVDT : Outport  Port=2
  GAS_LVDT : Outport  Port=3
  BF_LVDT : Outport  Port=4
  PF_OpLev : Outport  Port=5
  MN_PS : Outport  Port=6
  MN_OpLev : Outport  Port=7
  IM_PS : Outport  Port=8
  TM_OpLev : Outport  Port=9
  IM_OpLev : Outport  Port=10
  dispHL1-3 : Outport  Port=11
  dispHL2-3 : Outport  Port=12
  dispTM : Outport  Port=13
  dispBF : Outport  Port=14
  dispIP : Outport  Port=15
  wires:
  Suspension/1(dispGnd) -> [GND]
  Suspension/4(dispGAS) -> sMatrix_GAS_LVDT/1(dispGAS)
  Suspension/5(dispBF) -> dispBF/1, sMatrix_BF_LVDT/2(dispBF)
  sMatrix_IP_LVDT/1(IP_LVDT) -> IP_LVDT/1
  sMatrix_GAS_LVDT/1(GAS_LVDT) -> GAS_LVDT/1
  sMatrix_BF_LVDT/1(BF_LVDT) -> BF_LVDT/1
  Suspension/12(dispTM) -> sMatrix_TM_OpLev/1(dispTM), dispTM/1
  accGnd/1 -> Suspension/1(accGnd)
  actIP/1 -> Suspension/2(actIP)
  actGAS/1 -> aMatrix_GAS/1(aMat_in)
  actBF/1 -> aMatrix_BF/1(aMat_in)
  sMatrix_TM_OpLev/1(TM_OpLev) -> TM_OpLev/1
  aMatrix_GAS/1(actGAS) -> Suspension/3(actGAS)
  aMatrix_BF/1(actBF) -> Suspension/4(actBF)
  Suspension/6(dispPF) -> sMatrix_PF_OpLev/1(dispPF)
  sMatrix_PF_OpLev/1(PF_OpLev) -> PF_OpLev/1
  Suspension/7(dispMNR) -> sMatrix_MN_PS/1(dispMNR)
  Suspension/8(dispMN) -> sMatrix_MN_OpLev/1(dispMN), sMatrix_MN_PS/2(dispMN)
  sMatrix_MN_PS/1(MN_PS) -> MN_PS/1
  sMatrix_MN_OpLev/1(MN_OpLev) -> MN_OpLev/1
  Suspension/9(dispIR) -> sMatrix_IM_PS/1(dispIR)
  Suspension/10(dispIM) -> sMatrix_IM_OpLev/1(dispIM), sMatrix_IM_PS/2(dispIM)
  sMatrix_IM_PS/1(IM_PS) -> IM_PS/1
  Suspension/13(velTM) -> unused1/1
  aMatrix_MN/1(actMNR) -> Sum1/2
  aMatrix_MN/2(actMN) -> Suspension/6(actMN)
  actMN/1 -> aMatrix_MN/1(aMat_in)
  actIM/1 -> aMatrix_IM/1(aMat_in)
  aMatrix_IM/1(actIR) -> Suspension/7(actIR)
  aMatrix_IM/2(actIM) -> Suspension/8(actIM)
  actTM/1 -> aMatrix_TM/1(aMat_in)
  aMatrix_TM/1(actRM) -> Suspension/9(actRM)
  Sum/1 -> Suspension/10(actTM)
  aMatrix_TM/2(actTM) -> Sum/1
  forceTM/1 -> Sum/2
  Suspension/2(velIP) -> IP_GEO/1
  Sum1/1 -> Suspension/5(actMNR)
  forceMNR/1 -> Sum1/1
  Suspension/14(dispHL1-3) -> dispHL1-3/1
  Suspension/15(dispHL2-3) -> dispHL2-3/1
  Suspension/16(dispHLgnd1) -> unused2/1
  Suspension/17(dispHLgnd2) -> unused3/1
  accHLGnd1/1 -> Suspension/11(accHLGnd1)
  accHLGnd2/1 -> Suspension/12(accHLGnd2)
  Suspension/11(dispRM) -> unused/1
  [GND] -> sMatrix_IP_LVDT/1(dispGnd)
  [GND] -> sMatrix_BF_LVDT/1(dispGnd)
  sMatrix_IM_OpLev/1(IM_OpLev) -> IM_OpLev/1
  [GND] -> sMatrix_PF_OpLev/2(dispGND)
  [GND] -> sMatrix_MN_OpLev/2(dispGND)
  [GND] -> sMatrix_IM_OpLev/2(dispGND)
  [GND] -> sMatrix_TM_OpLev/2(dispGND)
  [GND] -> sMatrix_GAS_LVDT/2(dispGND)
  Suspension/3(dispIP) -> dispIP/1, sMatrix_IP_LVDT/2(dispIP)

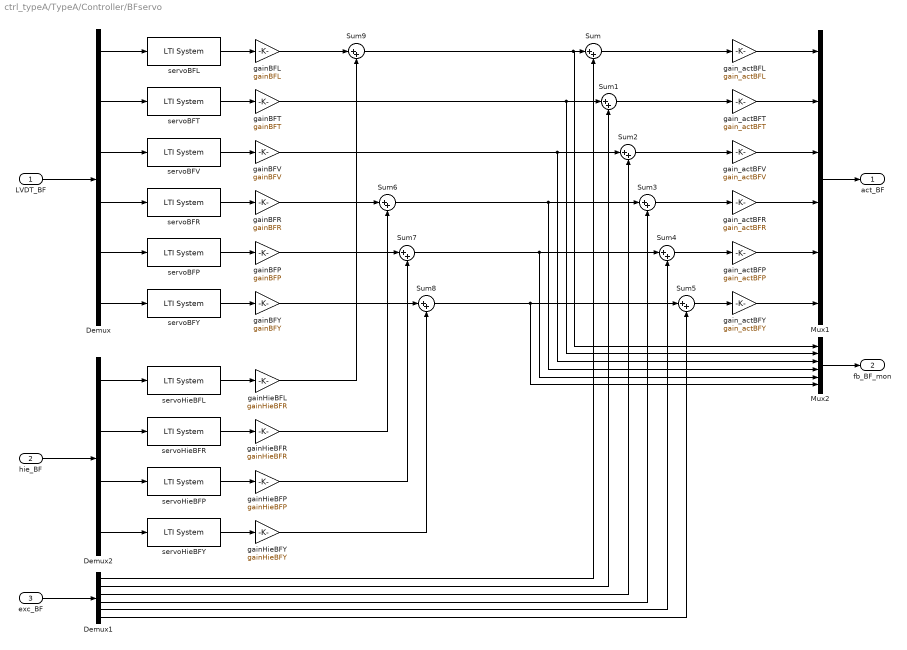
== system ctrl_typeA/TypeA/Controller/BFservo ==
  LVDT_BF : Inport
  hie_BF : Inport  Port=2
  exc_BF : Inport  Port=3
  Demux : Demux  Outputs=6
  Demux1 : Demux  Outputs=6
  Demux2 : Demux
  Mux1 : Mux  Inputs=6
  Mux2 : Mux  Inputs=6
  Sum{,1..9} (10 alike) : Sum  Inputs=|++
  gainBFL : Gain  Gain=gainBFL
  gainBFP : Gain  Gain=gainBFP
  gainBFR : Gain  Gain=gainBFR
  gainBFT : Gain  Gain=gainBFT
  gainBFV : Gain  Gain=gainBFV
  gainBFY : Gain  Gain=gainBFY
  gainHieBFL : Gain  Gain=gainHieBFR
  gainHieBFP : Gain  Gain=gainHieBFP
  gainHieBFR : Gain  Gain=gainHieBFR
  gainHieBFY : Gain  Gain=gainHieBFY
  gain_actBFL : Gain  Gain=gain_actBFL
  gain_actBFP : Gain  Gain=gain_actBFP
  gain_actBFR : Gain  Gain=gain_actBFR
  gain_actBFT : Gain  Gain=gain_actBFT
  gain_actBFV : Gain  Gain=gain_actBFV
  gain_actBFY : Gain  Gain=gain_actBFY
  servoBFL : cstblocks/LTI System  sys=servoBFL  IC=[]
  servoBFP : cstblocks/LTI System  sys=servoBFP  IC=[]
  servoBFR : cstblocks/LTI System  sys=servoBFR  IC=[]
  servoBFT : cstblocks/LTI System  sys=servoBFT  IC=[]
  servoBFV : cstblocks/LTI System  sys=servoBFV  IC=[]
  servoBFY : cstblocks/LTI System  sys=servoBFY  IC=[]
  servoHieBFL : cstblocks/LTI System  sys=servoHieBFL  IC=[]
  servoHieBFP : cstblocks/LTI System  sys=servoHieBFP  IC=[]
  servoHieBFR : cstblocks/LTI System  sys=servoHieBFR  IC=[]
  servoHieBFY : cstblocks/LTI System  sys=servoHieBFY  IC=[]
  act_BF : Outport
  fb_BF_mon : Outport  Port=2
  wires:
  LVDT_BF/1 -> Demux/1
  servoBFL/1 -> gainBFL/1
  servoBFT/1 -> gainBFT/1
  servoBFV/1 -> gainBFV/1
  Demux/1 -> servoBFL/1
  Demux/2 -> servoBFT/1
  Demux/3 -> servoBFV/1
  Sum9/1 -> Mux2/1, Sum/1
  gainBFT/1 -> Sum1/1, Mux2/2
  gainBFV/1 -> Sum2/1, Mux2/3
  exc_BF/1 -> Demux1/1
  Sum1/1 -> gain_actBFT/1
  Sum2/1 -> gain_actBFV/1
  Sum/1 -> gain_actBFL/1
  Mux1/1 -> act_BF/1
  Mux2/1 -> fb_BF_mon/1
  Demux1/3 -> Sum2/2
  Demux1/2 -> Sum1/2
  Demux1/1 -> Sum/2
  servoBFR/1 -> gainBFR/1
  servoBFP/1 -> gainBFP/1
  Sum6/1 -> Sum3/1, Mux2/4
  Sum7/1 -> Sum4/1, Mux2/5
  Demux/4 -> servoBFR/1
  Demux/5 -> servoBFP/1
  Demux1/4 -> Sum3/2
  Demux1/5 -> Sum4/2
  Sum3/1 -> gain_actBFR/1
  Sum4/1 -> gain_actBFP/1
  servoBFY/1 -> gainBFY/1
  Sum8/1 -> Sum5/1, Mux2/6
  Demux/6 -> servoBFY/1
  Sum5/1 -> gain_actBFY/1
  gain_actBFV/1 -> Mux1/3
  gain_actBFY/1 -> Mux1/6
  gain_actBFR/1 -> Mux1/4
  gain_actBFT/1 -> Mux1/2
  gain_actBFL/1 -> Mux1/1
  gain_actBFP/1 -> Mux1/5
  servoHieBFR/1 -> gainHieBFR/1
  servoHieBFP/1 -> gainHieBFP/1
  servoHieBFY/1 -> gainHieBFY/1
  hie_BF/1 -> Demux2/1
  gainBFR/1 -> Sum6/1
  gainBFP/1 -> Sum7/1
  gainBFY/1 -> Sum8/1
  gainHieBFR/1 -> Sum6/2
  gainHieBFP/1 -> Sum7/2
  gainHieBFY/1 -> Sum8/2
  Demux2/1 -> servoHieBFL/1
  Demux2/2 -> servoHieBFR/1
  Demux2/3 -> servoHieBFP/1
  Demux2/4 -> servoHieBFY/1
  servoHieBFL/1 -> gainHieBFL/1
  gainBFL/1 -> Sum9/1
  gainHieBFL/1 -> Sum9/2
  Demux1/6 -> Sum5/2

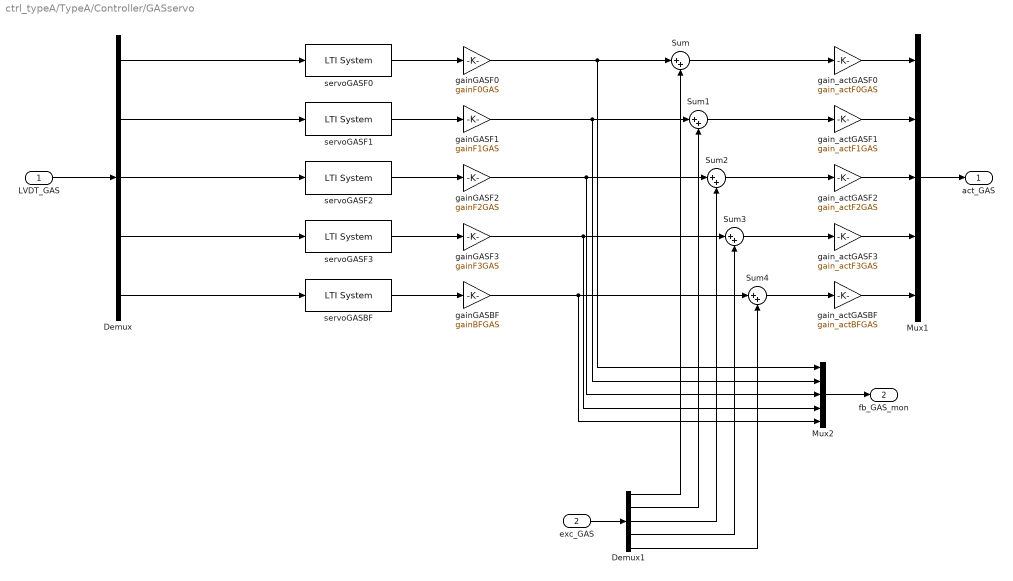
== system ctrl_typeA/TypeA/Controller/GASservo ==
  LVDT_GAS : Inport
  exc_GAS : Inport  Port=2
  Demux : Demux  Outputs=5
  Demux1 : Demux  Outputs=5
  Mux1 : Mux  Inputs=5
  Mux2 : Mux  Inputs=5
  Sum{,1..4} (5 alike) : Sum  Inputs=|++
  gainGASBF : Gain  Gain=gainBFGAS
  gainGASF0 : Gain  Gain=gainF0GAS
  gainGASF1 : Gain  Gain=gainF1GAS
  gainGASF2 : Gain  Gain=gainF2GAS
  gainGASF3 : Gain  Gain=gainF3GAS
  gain_actGASBF : Gain  Gain=gain_actBFGAS
  gain_actGASF0 : Gain  Gain=gain_actF0GAS
  gain_actGASF1 : Gain  Gain=gain_actF1GAS
  gain_actGASF2 : Gain  Gain=gain_actF2GAS
  gain_actGASF3 : Gain  Gain=gain_actF3GAS
  servoGASBF : cstblocks/LTI System  sys=servoBFGAS  IC=[]
  servoGASF0 : cstblocks/LTI System  sys=servoF0GAS  IC=[]
  servoGASF1 : cstblocks/LTI System  sys=servoF1GAS  IC=[]
  servoGASF2 : cstblocks/LTI System  sys=servoF2GAS  IC=[]
  servoGASF3 : cstblocks/LTI System  sys=servoF3GAS  IC=[]
  act_GAS : Outport
  fb_GAS_mon : Outport  Port=2
  wires:
  LVDT_GAS/1 -> Demux/1
  servoGASF0/1 -> gainGASF0/1
  servoGASF1/1 -> gainGASF1/1
  servoGASF2/1 -> gainGASF2/1
  Demux/1 -> servoGASF0/1
  Demux/2 -> servoGASF1/1
  Demux/3 -> servoGASF2/1
  gainGASF0/1 -> Sum/1, Mux2/1
  gainGASF1/1 -> Sum1/1, Mux2/2
  gainGASF2/1 -> Sum2/1, Mux2/3
  exc_GAS/1 -> Demux1/1
  Sum1/1 -> gain_actGASF1/1
  Sum2/1 -> gain_actGASF2/1
  Sum/1 -> gain_actGASF0/1
  Mux1/1 -> act_GAS/1
  Mux2/1 -> fb_GAS_mon/1
  Demux1/3 -> Sum2/2
  Demux1/2 -> Sum1/2
  Demux1/1 -> Sum/2
  servoGASF3/1 -> gainGASF3/1
  servoGASBF/1 -> gainGASBF/1
  gainGASF3/1 -> Sum3/1, Mux2/4
  gainGASBF/1 -> Sum4/1, Mux2/5
  Demux/4 -> servoGASF3/1
  Demux/5 -> servoGASBF/1
  Demux1/4 -> Sum3/2
  Demux1/5 -> Sum4/2
  Sum3/1 -> gain_actGASF3/1
  Sum4/1 -> gain_actGASBF/1
  gain_actGASF0/1 -> Mux1/1
  gain_actGASF2/1 -> Mux1/3
  gain_actGASF1/1 -> Mux1/2
  gain_actGASF3/1 -> Mux1/4
  gain_actGASBF/1 -> Mux1/5

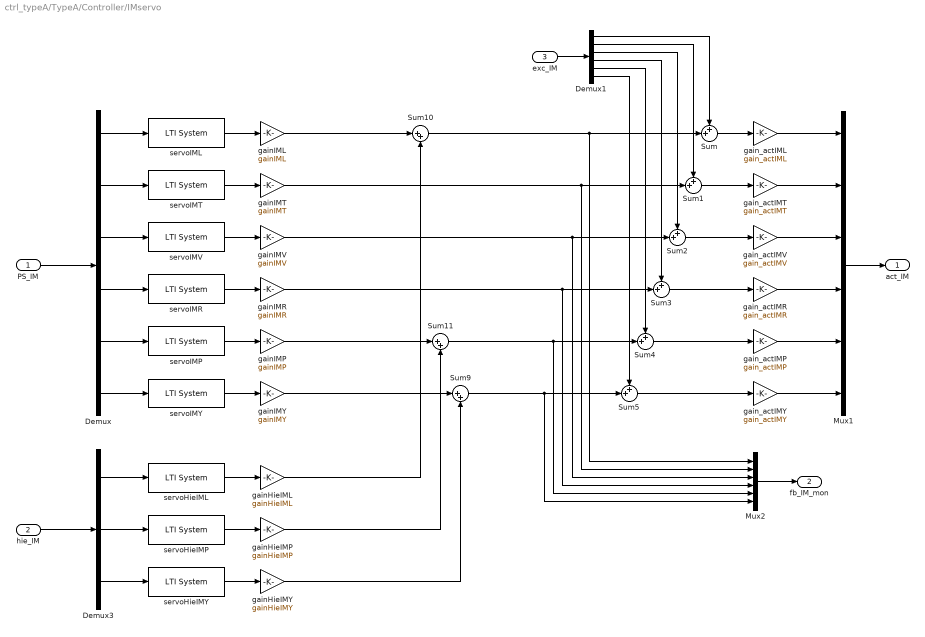
== system ctrl_typeA/TypeA/Controller/IMservo ==
  PS_IM : Inport
  hie_IM : Inport  Port=2
  exc_IM : Inport  Port=3
  Demux : Demux  Outputs=6
  Demux1 : Demux  Outputs=6
  Demux3 : Demux  Outputs=3
  Mux1 : Mux  Inputs=6
  Mux2 : Mux  Inputs=6
  Sum{,1..5} (6 alike) : Sum  Inputs=++|
  Sum10 : Sum  Inputs=|++
  Sum11 : Sum  Inputs=|++
  Sum9 : Sum  Inputs=|++
  gainHieIML : Gain  Gain=gainHieIML
  gainHieIMP : Gain  Gain=gainHieIMP
  gainHieIMY : Gain  Gain=gainHieIMY
  gainIML : Gain  Gain=gainIML
  gainIMP : Gain  Gain=gainIMP
  gainIMR : Gain  Gain=gainIMR
  gainIMT : Gain  Gain=gainIMT
  gainIMV : Gain  Gain=gainIMV
  gainIMY : Gain  Gain=gainIMY
  gain_actIML : Gain  Gain=gain_actIML
  gain_actIMP : Gain  Gain=gain_actIMP
  gain_actIMR : Gain  Gain=gain_actIMR
  gain_actIMT : Gain  Gain=gain_actIMT
  gain_actIMV : Gain  Gain=gain_actIMV
  gain_actIMY : Gain  Gain=gain_actIMY
  servoHieIML : cstblocks/LTI System  sys=servoHieIML  IC=[]
  servoHieIMP : cstblocks/LTI System  sys=servoHieIMP  IC=[]
  servoHieIMY : cstblocks/LTI System  sys=servoHieIMY  IC=[]
  servoIML : cstblocks/LTI System  sys=servoIML  IC=[]
  servoIMP : cstblocks/LTI System  sys=servoIMP  IC=[]
  servoIMR : cstblocks/LTI System  sys=servoIMR  IC=[]
  servoIMT : cstblocks/LTI System  sys=servoIMT  IC=[]
  servoIMV : cstblocks/LTI System  sys=servoIMV  IC=[]
  servoIMY : cstblocks/LTI System  sys=servoIMY  IC=[]
  act_IM : Outport
  fb_IM_mon : Outport  Port=2
  wires:
  PS_IM/1 -> Demux/1
  servoIML/1 -> gainIML/1
  servoIMT/1 -> gainIMT/1
  servoIMV/1 -> gainIMV/1
  Demux/1 -> servoIML/1
  Demux/2 -> servoIMT/1
  Demux/3 -> servoIMV/1
  Sum10/1 -> Sum/2, Mux2/1
  gainIMT/1 -> Sum1/2, Mux2/2
  gainIMV/1 -> Sum2/2, Mux2/3
  exc_IM/1 -> Demux1/1
  Sum1/1 -> gain_actIMT/1
  Sum2/1 -> gain_actIMV/1
  Sum/1 -> gain_actIML/1
  Mux1/1 -> act_IM/1
  Mux2/1 -> fb_IM_mon/1
  Demux1/3 -> Sum2/1
  Demux1/2 -> Sum1/1
  Demux1/1 -> Sum/1
  servoIMR/1 -> gainIMR/1
  servoIMP/1 -> gainIMP/1
  gainIMR/1 -> Sum3/2, Mux2/4
  Sum11/1 -> Sum4/2, Mux2/5
  Demux/4 -> servoIMR/1
  Demux/5 -> servoIMP/1
  Demux1/4 -> Sum3/1
  Demux1/5 -> Sum4/1
  Sum3/1 -> gain_actIMR/1
  Sum4/1 -> gain_actIMP/1
  servoIMY/1 -> gainIMY/1
  Sum9/1 -> Sum5/2, Mux2/6
  Demux/6 -> servoIMY/1
  Sum5/1 -> gain_actIMY/1
  Demux1/6 -> Sum5/1
  gain_actIMV/1 -> Mux1/3
  gain_actIMY/1 -> Mux1/6
  gain_actIMR/1 -> Mux1/4
  gain_actIMT/1 -> Mux1/2
  gain_actIML/1 -> Mux1/1
  gain_actIMP/1 -> Mux1/5
  servoHieIML/1 -> gainHieIML/1
  servoHieIMP/1 -> gainHieIMP/1
  servoHieIMY/1 -> gainHieIMY/1
  hie_IM/1 -> Demux3/1
  Demux3/1 -> servoHieIML/1
  Demux3/2 -> servoHieIMP/1
  Demux3/3 -> servoHieIMY/1
  gainIML/1 -> Sum10/1
  gainIMP/1 -> Sum11/1
  gainHieIML/1 -> Sum10/2
  gainHieIMP/1 -> Sum11/2
  gainHieIMY/1 -> Sum9/2
  gainIMY/1 -> Sum9/1

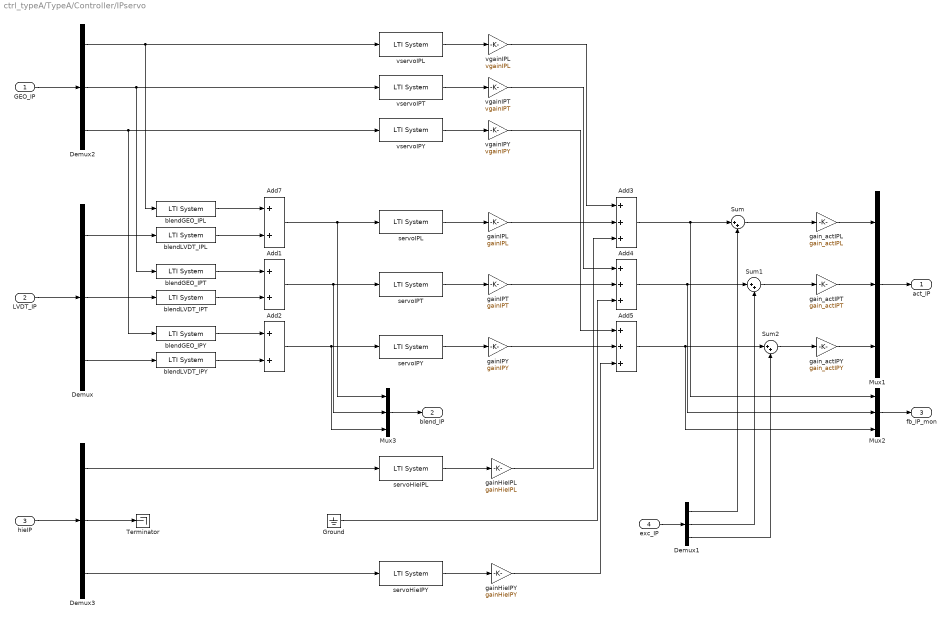
== system ctrl_typeA/TypeA/Controller/IPservo ==
  GEO_IP : Inport
  LVDT_IP : Inport  Port=2
  hieIP : Inport  Port=3
  exc_IP : Inport  Port=4
  Add1 : Sum
  Add2 : Sum
  Add3 : Sum  Inputs=+++
  Add4 : Sum  Inputs=+++
  Add5 : Sum  Inputs=+++
  Add7 : Sum
  Demux{,1..3} (4 alike) : Demux  Outputs=3
  Ground : Ground
  Mux1 : Mux  Inputs=3
  Mux2 : Mux  Inputs=3
  Mux3 : Mux  Inputs=3
  Sum : Sum  Inputs=|++
  Sum1 : Sum  Inputs=|++
  Sum2 : Sum  Inputs=|++
  Terminator : Terminator
  blendGEO_IPL : cstblocks/LTI System  sys=blendGEO_IPL  IC=[]
  blendGEO_IPT : cstblocks/LTI System  sys=blendGEO_IPT  IC=[]
  blendGEO_IPY : cstblocks/LTI System  sys=blendGEO_IPY  IC=[]
  blendLVDT_IPL : cstblocks/LTI System  sys=blendLVDT_IPL  IC=[]
  blendLVDT_IPT : cstblocks/LTI System  sys=blendLVDT_IPT  IC=[]
  blendLVDT_IPY : cstblocks/LTI System  sys=blendLVDT_IPY  IC=[]
  gainHieIPL : Gain  Gain=gainHieIPL
  gainHieIPY : Gain  Gain=gainHieIPY
  gainIPL : Gain  Gain=gainIPL
  gainIPT : Gain  Gain=gainIPT
  gainIPY : Gain  Gain=gainIPY
  gain_actIPL : Gain  Gain=gain_actIPL
  gain_actIPT : Gain  Gain=gain_actIPT
  gain_actIPY : Gain  Gain=gain_actIPY
  servoHieIPL : cstblocks/LTI System  sys=servoHieIPL  IC=[]
  servoHieIPY : cstblocks/LTI System  sys=servoHieIPY  IC=[]
  servoIPL : cstblocks/LTI System  sys=servoIPL  IC=[]
  servoIPT : cstblocks/LTI System  sys=servoIPT  IC=[]
  servoIPY : cstblocks/LTI System  sys=servoIPY  IC=[]
  vgainIPL : Gain  Gain=vgainIPL
  vgainIPT : Gain  Gain=vgainIPT
  vgainIPY : Gain  Gain=vgainIPY
  vservoIPL : cstblocks/LTI System  sys=vservoIPL  IC=[]
  vservoIPT : cstblocks/LTI System  sys=vservoIPT  IC=[]
  vservoIPY : cstblocks/LTI System  sys=vservoIPY  IC=[]
  act_IP : Outport
  blend_IP : Outport  Port=2
  fb_IP_mon : Outport  Port=3
  wires:
  LVDT_IP/1 -> Demux/1
  servoIPL/1 -> gainIPL/1
  servoIPT/1 -> gainIPT/1
  servoIPY/1 -> gainIPY/1
  Add3/1 -> Sum/1, Mux2/1
  Add4/1 -> Sum1/1, Mux2/2
  Add5/1 -> Sum2/1, Mux2/3
  exc_IP/1 -> Demux1/1
  Sum1/1 -> gain_actIPT/1
  Sum2/1 -> gain_actIPY/1
  Sum/1 -> gain_actIPL/1
  Mux1/1 -> act_IP/1
  Mux2/1 -> fb_IP_mon/1
  Demux1/3 -> Sum2/2
  Demux1/2 -> Sum1/2
  Demux1/1 -> Sum/2
  gain_actIPT/1 -> Mux1/2
  gain_actIPL/1 -> Mux1/1
  gain_actIPY/1 -> Mux1/3
  Demux/2 -> blendLVDT_IPT/1
  Demux/3 -> blendLVDT_IPY/1
  Demux/1 -> blendLVDT_IPL/1
  GEO_IP/1 -> Demux2/1
  Demux2/2 -> vservoIPT/1, blendGEO_IPT/1
  Demux2/3 -> vservoIPY/1, blendGEO_IPY/1
  Demux2/1 -> vservoIPL/1, blendGEO_IPL/1
  Add7/1 -> Mux3/1, servoIPL/1
  Add1/1 -> Mux3/2, servoIPT/1
  Add2/1 -> Mux3/3, servoIPY/1
  blendGEO_IPL/1 -> Add7/1
  blendGEO_IPT/1 -> Add1/1
  blendGEO_IPY/1 -> Add2/1
  blendLVDT_IPL/1 -> Add7/2
  blendLVDT_IPT/1 -> Add1/2
  blendLVDT_IPY/1 -> Add2/2
  Mux3/1 -> blend_IP/1
  vservoIPL/1 -> vgainIPL/1
  vservoIPT/1 -> vgainIPT/1
  vservoIPY/1 -> vgainIPY/1
  gainIPY/1 -> Add5/2
  gainIPT/1 -> Add4/2
  gainIPL/1 -> Add3/2
  vgainIPL/1 -> Add3/1
  vgainIPT/1 -> Add4/1
  vgainIPY/1 -> Add5/1
  servoHieIPL/1 -> gainHieIPL/1
  servoHieIPY/1 -> gainHieIPY/1
  hieIP/1 -> Demux3/1
  Demux3/1 -> servoHieIPL/1
  Demux3/3 -> servoHieIPY/1
  gainHieIPL/1 -> Add3/3
  gainHieIPY/1 -> Add5/3
  Demux3/2 -> Terminator/1
  Ground/1 -> Add4/3

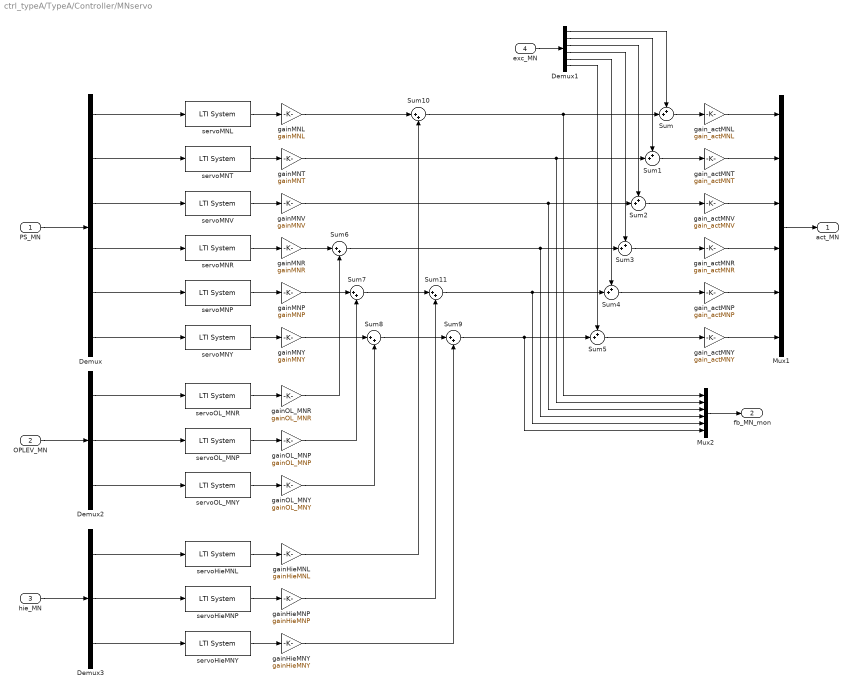
== system ctrl_typeA/TypeA/Controller/MNservo ==
  PS_MN : Inport
  OPLEV_MN : Inport  Port=2
  hie_MN : Inport  Port=3
  exc_MN : Inport  Port=4
  Demux : Demux  Outputs=6
  Demux1 : Demux  Outputs=6
  Demux2 : Demux  Outputs=3
  Demux3 : Demux  Outputs=3
  Mux1 : Mux  Inputs=6
  Mux2 : Mux  Inputs=6
  Sum{,1..5} (6 alike) : Sum  Inputs=++|
  Sum{6..11} (6 alike) : Sum  Inputs=|++
  gainHieMNL : Gain  Gain=gainHieMNL
  gainHieMNP : Gain  Gain=gainHieMNP
  gainHieMNY : Gain  Gain=gainHieMNY
  gainMNL : Gain  Gain=gainMNL
  gainMNP : Gain  Gain=gainMNP
  gainMNR : Gain  Gain=gainMNR
  gainMNT : Gain  Gain=gainMNT
  gainMNV : Gain  Gain=gainMNV
  gainMNY : Gain  Gain=gainMNY
  gainOL_MNP : Gain  Gain=gainOL_MNP
  gainOL_MNR : Gain  Gain=gainOL_MNR
  gainOL_MNY : Gain  Gain=gainOL_MNY
  gain_actMNL : Gain  Gain=gain_actMNL
  gain_actMNP : Gain  Gain=gain_actMNP
  gain_actMNR : Gain  Gain=gain_actMNR
  gain_actMNT : Gain  Gain=gain_actMNT
  gain_actMNV : Gain  Gain=gain_actMNV
  gain_actMNY : Gain  Gain=gain_actMNY
  servoHieMNL : cstblocks/LTI System  sys=servoHieMNL  IC=[]
  servoHieMNP : cstblocks/LTI System  sys=servoHieMNP  IC=[]
  servoHieMNY : cstblocks/LTI System  sys=servoHieMNY  IC=[]
  servoMNL : cstblocks/LTI System  sys=servoMNL  IC=[]
  servoMNP : cstblocks/LTI System  sys=servoMNP  IC=[]
  servoMNR : cstblocks/LTI System  sys=servoMNR  IC=[]
  servoMNT : cstblocks/LTI System  sys=servoMNT  IC=[]
  servoMNV : cstblocks/LTI System  sys=servoMNV  IC=[]
  servoMNY : cstblocks/LTI System  sys=servoMNY  IC=[]
  servoOL_MNP : cstblocks/LTI System  sys=servoOL_MNP  IC=[]
  servoOL_MNR : cstblocks/LTI System  sys=servoOL_MNR  IC=[]
  servoOL_MNY : cstblocks/LTI System  sys=servoOL_MNY  IC=[]
  act_MN : Outport
  fb_MN_mon : Outport  Port=2
  wires:
  PS_MN/1 -> Demux/1
  servoMNL/1 -> gainMNL/1
  servoMNT/1 -> gainMNT/1
  servoMNV/1 -> gainMNV/1
  Demux/1 -> servoMNL/1
  Demux/2 -> servoMNT/1
  Demux/3 -> servoMNV/1
  Sum10/1 -> Sum/2, Mux2/1
  gainMNT/1 -> Sum1/2, Mux2/2
  gainMNV/1 -> Sum2/2, Mux2/3
  exc_MN/1 -> Demux1/1
  Sum1/1 -> gain_actMNT/1
  Sum2/1 -> gain_actMNV/1
  Sum/1 -> gain_actMNL/1
  Mux1/1 -> act_MN/1
  Mux2/1 -> fb_MN_mon/1
  Demux1/3 -> Sum2/1
  Demux1/2 -> Sum1/1
  Demux1/1 -> Sum/1
  servoMNR/1 -> gainMNR/1
  servoMNP/1 -> gainMNP/1
  Sum6/1 -> Sum3/2, Mux2/4
  Sum11/1 -> Sum4/2, Mux2/5
  Demux/4 -> servoMNR/1
  Demux/5 -> servoMNP/1
  Demux1/4 -> Sum3/1
  Demux1/5 -> Sum4/1
  Sum3/1 -> gain_actMNR/1
  Sum4/1 -> gain_actMNP/1
  servoMNY/1 -> gainMNY/1
  Sum9/1 -> Sum5/2, Mux2/6
  Demux/6 -> servoMNY/1
  Sum5/1 -> gain_actMNY/1
  Demux1/6 -> Sum5/1
  gain_actMNV/1 -> Mux1/3
  gain_actMNY/1 -> Mux1/6
  gain_actMNR/1 -> Mux1/4
  gain_actMNT/1 -> Mux1/2
  gain_actMNL/1 -> Mux1/1
  gain_actMNP/1 -> Mux1/5
  servoHieMNL/1 -> gainHieMNL/1
  servoHieMNP/1 -> gainHieMNP/1
  servoHieMNY/1 -> gainHieMNY/1
  servoOL_MNR/1 -> gainOL_MNR/1
  servoOL_MNP/1 -> gainOL_MNP/1
  servoOL_MNY/1 -> gainOL_MNY/1
  OPLEV_MN/1 -> Demux2/1
  hie_MN/1 -> Demux3/1
  Demux2/1 -> servoOL_MNR/1
  Demux2/2 -> servoOL_MNP/1
  Demux2/3 -> servoOL_MNY/1
  Demux3/1 -> servoHieMNL/1
  gainMNR/1 -> Sum6/1
  gainMNP/1 -> Sum7/1
  gainMNY/1 -> Sum8/1
  gainOL_MNR/1 -> Sum6/2
  gainOL_MNP/1 -> Sum7/2
  gainOL_MNY/1 -> Sum8/2
  gainMNL/1 -> Sum10/1
  Sum7/1 -> Sum11/1
  gainHieMNL/1 -> Sum10/2
  gainHieMNP/1 -> Sum11/2
  gainHieMNY/1 -> Sum9/2
  Sum8/1 -> Sum9/1
  Demux3/2 -> servoHieMNP/1
  Demux3/3 -> servoHieMNY/1

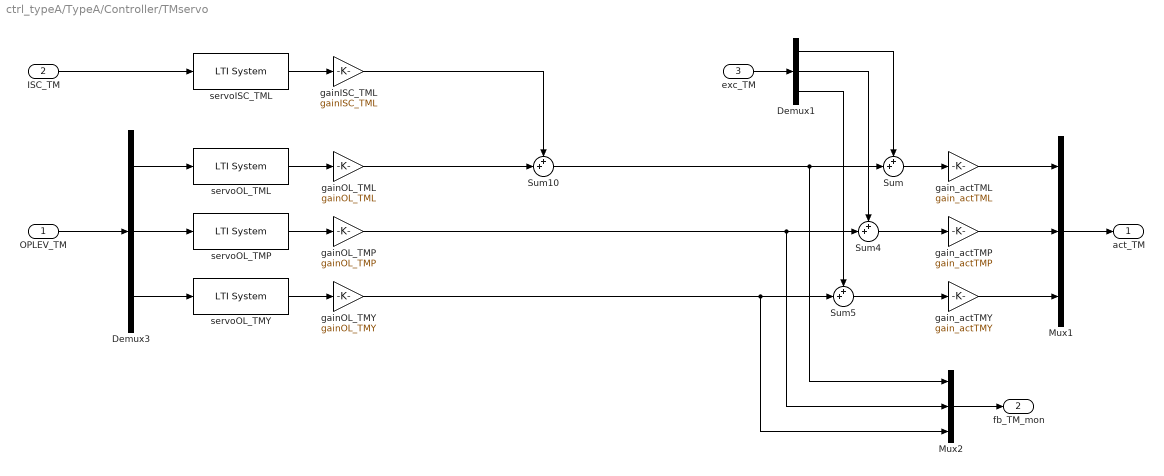
== system ctrl_typeA/TypeA/Controller/TMservo ==
  OPLEV_TM : Inport
  ISC_TM : Inport  Port=2
  exc_TM : Inport  Port=3
  Demux1 : Demux  Outputs=3
  Demux3 : Demux  Outputs=3
  Mux1 : Mux  Inputs=3
  Mux2 : Mux  Inputs=3
  Sum{,4..5,10} (4 alike) : Sum  Inputs=++|
  gainISC_TML : Gain  Gain=gainISC_TML
  gainOL_TML : Gain  Gain=gainOL_TML
  gainOL_TMP : Gain  Gain=gainOL_TMP
  gainOL_TMY : Gain  Gain=gainOL_TMY
  gain_actTML : Gain  Gain=gain_actTML
  gain_actTMP : Gain  Gain=gain_actTMP
  gain_actTMY : Gain  Gain=gain_actTMY
  servoISC_TML : cstblocks/LTI System  sys=servoISC_TML  IC=[]
  servoOL_TML : cstblocks/LTI System  sys=servoOL_TML  IC=[]
  servoOL_TMP : cstblocks/LTI System  sys=servoOL_TMP  IC=[]
  servoOL_TMY : cstblocks/LTI System  sys=servoOL_TMY  IC=[]
  act_TM : Outport
  fb_TM_mon : Outport  Port=2
  wires:
  Sum10/1 -> Sum/2, Mux2/1
  exc_TM/1 -> Demux1/1
  Sum/1 -> gain_actTML/1
  Mux1/1 -> act_TM/1
  Mux2/1 -> fb_TM_mon/1
  Demux1/1 -> Sum/1
  Sum4/1 -> gain_actTMP/1
  Sum5/1 -> gain_actTMY/1
  gain_actTML/1 -> Mux1/1
  servoOL_TMP/1 -> gainOL_TMP/1
  servoOL_TMY/1 -> gainOL_TMY/1
  OPLEV_TM/1 -> Demux3/1
  Demux3/2 -> servoOL_TMP/1
  Demux3/3 -> servoOL_TMY/1
  gainOL_TMP/1 -> Mux2/2, Sum4/2
  gainOL_TMY/1 -> Mux2/3, Sum5/2
  Demux1/2 -> Sum4/1
  Demux1/3 -> Sum5/1
  gain_actTMP/1 -> Mux1/2
  gain_actTMY/1 -> Mux1/3
  servoISC_TML/1 -> gainISC_TML/1
  ISC_TM/1 -> servoISC_TML/1
  Demux3/1 -> servoOL_TML/1
  servoOL_TML/1 -> gainOL_TML/1
  gainOL_TML/1 -> Sum10/2
  gainISC_TML/1 -> Sum10/1

== system ctrl_typeA/TypeA/Controller/sum ==
  localTM : Inport
  globalISC : Inport  Port=2
  Demux4 : Demux  Outputs=3
  Mux3 : Mux  Inputs=3
  Sum : Sum  Inputs=++|
  toUpperStage : Outport
  wires:
  localTM/1 -> Demux4/1
  Mux3/1 -> toUpperStage/1
  Demux4/1 -> Sum/2  "L"
  Demux4/2 -> Mux3/2  "P"
  Demux4/3 -> Mux3/3  "Y"
  globalISC/1 -> Sum/1
  Sum/1 -> Mux3/1

== system ctrl_typeA/TypeA/Controller/sum1 ==
  fromPF : Inport
  fromTM : Inport  Port=2
  Demux1 : Demux  Outputs=3
  Demux4 : Demux  Outputs=3
  Mux3 : Mux
  Sum : Sum  Inputs=++|
  Sum1 : Sum  Inputs=++|
  toBF : Outport
  wires:
  fromTM/1 -> Demux4/1
  Mux3/1 -> toBF/1
  Demux4/2 -> Sum/2  "P"
  Demux4/3 -> Sum1/2  "Y"
  fromPF/1 -> Demux1/1
  Sum1/1 -> Mux3/4
  Demux4/1 -> Mux3/1  "L"
  Demux1/2 -> Sum/1  "P"
  Demux1/3 -> Sum1/1  "Y"
  Sum/1 -> Mux3/3
  Demux1/1 -> Mux3/2  "R"
